simulink model "te_controller"  (R2013b)
settings: Solver=ode5  SolverMode=SingleTasking  StartTime=0.0  StopTime=15  FixedStep=Ts_base  MaxStep=Ts_base  MinStep=1e-6  RelTol=1e-6
InitFcn:
  | global model_type
  | model_type = 1  % plant and controller
  | 
  | init_model
StopFcn:
  | %TEplot
libraries: TEsim_utils x1
settings Model: Creator=rnc4  LastModifiedBy=rnc4
settings DataIOCC: LimitDataPoints=off  LoadInitialState=on  SaveFinalState=on  SaveFormat=Structure  SignalLoggingSaveFormat=ModelDataLogs  SaveOutput=off  SaveTime=off  SignalLoggingName=sigsOut
settings OptimizationCC: InitFltsAndDblsToZero=on
settings DebuggingCC: SaveWithParameterizedLinksMsg=none  SignalResolutionControl=TryResolveAllWithWarning  SolverPrmCheckMsg=none  MultiTaskDSMMsg=warning  MultiTaskCondExecSysMsg=none  FcnCallInpInsideContextMsg=UseLocalSettings  StrictBusMsg=None
settings HardwareCC: TargetUnknown=on
settings RTWCC: IncludeERTFirstTime=on
settings GRTTargetCC: TargetFcnLib=ansi_tfl_tmw.mat  CodeReplacementLibrary=None  CombineOutputUpdateFcns=off  CPPClassGenCompliant=on  GRTInterface=on

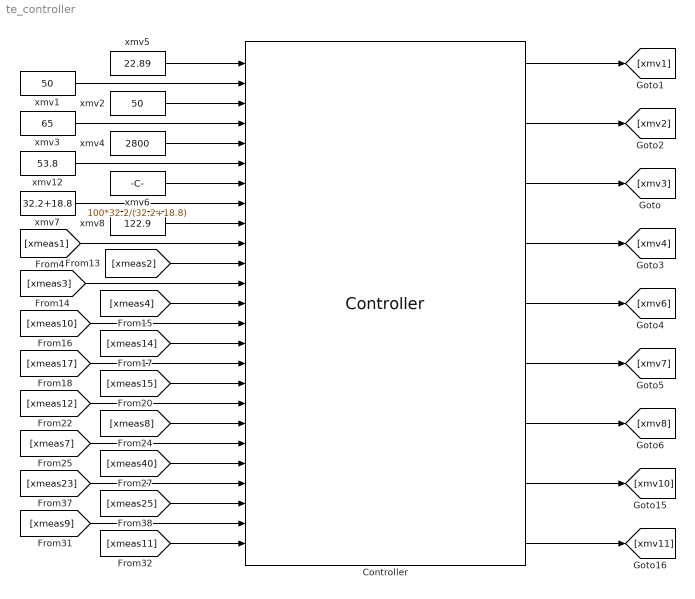
== system te_controller ==
  Controller : TEsim_utils/TEsim/Controller
  xmv1 : Constant  Value=50
  xmv12 : Constant  Value=53.8
  xmv2 : Constant  Value=50
  xmv3 : Constant  Value=65
  xmv4 : Constant  Value=2800
  xmv5 : Constant  Value=22.89
  xmv6 : Constant  Value=100*32.2/(32.2+18.8)
  xmv7 : Constant  Value=32.2+18.8
  xmv8 : Constant  Value=122.9
  wires:
  xmv8/1 -> Controller/9
  xmv7/1 -> Controller/8
  xmv6/1 -> Controller/7
  xmv12/1 -> Controller/6
  xmv4/1 -> Controller/5
  xmv3/1 -> Controller/4
  xmv2/1 -> Controller/3
  xmv1/1 -> Controller/2
  xmv5/1 -> Controller/1
  [xmeas1] -> Controller/10
  [xmeas2] -> Controller/11
  [xmeas3] -> Controller/12
  [xmeas4] -> Controller/13
  [xmeas10] -> Controller/14
  [xmeas14] -> Controller/15
  [xmeas17] -> Controller/16
  [xmeas15] -> Controller/17
  [xmeas12] -> Controller/18
  [xmeas8] -> Controller/19
  [xmeas7] -> Controller/20
  [xmeas40] -> Controller/21
  [xmeas23] -> Controller/22
  [xmeas25] -> Controller/23
  [xmeas9] -> Controller/24
  [xmeas11] -> Controller/25
  Controller/1 -> [xmv1]
  Controller/2 -> [xmv2]
  Controller/3 -> [xmv3]
  Controller/4 -> [xmv4]
  Controller/5 -> [xmv6]
  Controller/6 -> [xmv7]
  Controller/7 -> [xmv8]
  Controller/8 -> [xmv10]
  Controller/9 -> [xmv11]
